simulink model "DC_Model2"  (R2024b)
settings: Solver=VariableStepAuto  StartTime=0.0  StopTime=10  RelTol=1e-6
model workspace (MAT data in the model file):
  B = 0.1
  J = 0.01
  Ke = 0.01
  Kt = 0.01
  L = 0.5
  Req = 1
  Vbat = 24
settings Model: Creator=khalid  LastModifiedBy=khalidwaleed

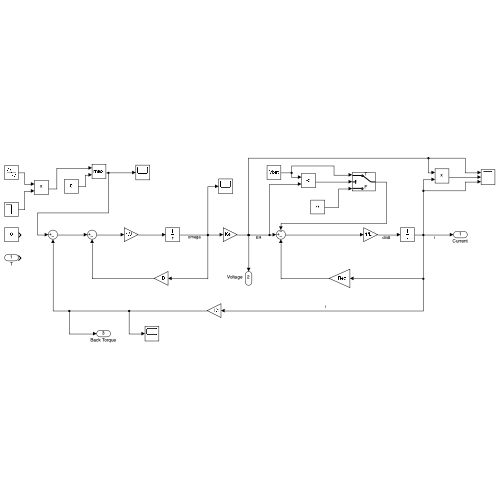
[thumbnail: Simulink's stored preview of the top-level diagram]
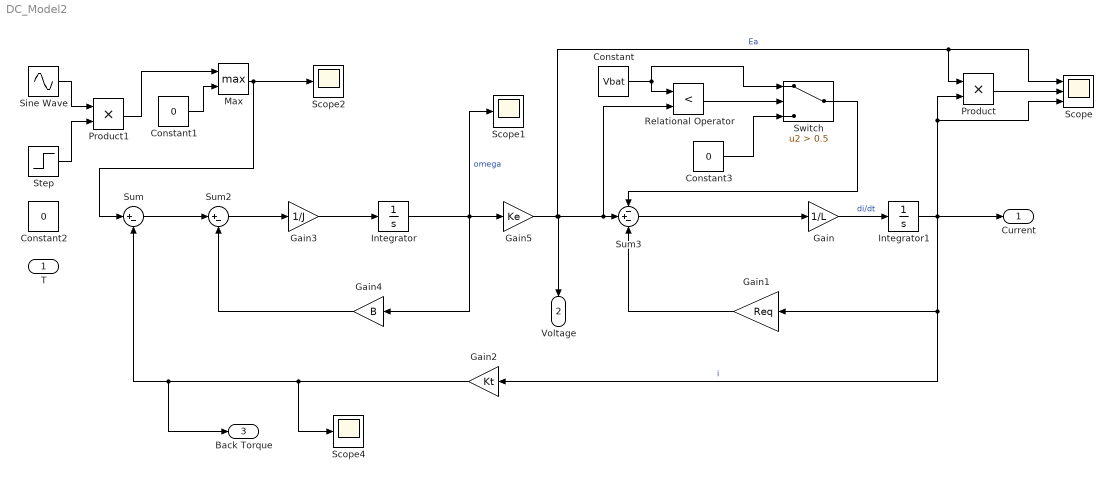
== system DC_Model2 ==
  T : Inport
  Constant : Constant  Value=Vbat
  Constant1 : Constant  Value=0
  Constant2 : Constant  Value=0
  Constant3 : Constant  Value=0
  Gain : Gain  Gain=1/L
  Gain1 : Gain  Gain=Req
  Gain2 : Gain  Gain=Kt
  Gain3 : Gain  Gain=1/J
  Gain4 : Gain  Gain=B
  Gain5 : Gain  Gain=Ke
  Integrator : Integrator
  Integrator1 : Integrator
  Max : MinMax  Function=max  Inputs=2
  Product : Product
  Product1 : Product
  Relational Operator : RelationalOperator  Operator=<  OutDataTypeStr=boolean  RndMeth=Simplest  InputSameDT=off
  Scope : Scope  NumInputPorts=3
  Scope1 : Scope
  Scope2 : Scope
  Scope4 : Scope
  Sine Wave : Sin  Amplitude=1e3  Frequency=20  SampleTime=0
  Step : Step  Time=5  Before=1  After=0  SampleTime=0
  Sum : Sum  Inputs=|+-
  Sum2 : Sum  Inputs=|+-
  Sum3 : Sum  Inputs=-+-
  Switch : Switch  Criteria=u2 > Threshold  Threshold=0.5  SaturateOnIntegerOverflow=off  InputSameDT=off
  Current : Outport
  Voltage : Outport  Port=2
  Back Torque : Outport  Port=3
  wires:
  Gain4/1 -> Sum2/2
  Gain3/1 -> Integrator/1
  Integrator/1 -> Gain5/1, Gain4/1, Scope1/1  "omega"
  Gain2/1 -> Scope4/1, Back Torque/1, Sum/2
  Integrator1/1 -> Gain1/1, Gain2/1, Product/2, Scope/3, Current/1  "i"
  Sum/1 -> Sum2/1
  Gain5/1 -> Relational Operator/2, Sum3/2, Voltage/1, Product/1, Scope/1  "Ea"
  Gain/1 -> Integrator1/1  "di/dt"
  Sum2/1 -> Gain3/1
  Product/1 -> Scope/2
  Sine Wave/1 -> Product1/1
  Step/1 -> Product1/2
  Constant1/1 -> Max/2
  Product1/1 -> Max/1
  Max/1 -> Sum/1, Scope2/1
  Gain1/1 -> Sum3/3
  Sum3/1 -> Gain/1
  Constant/1 -> Switch/1, Relational Operator/1
  Constant3/1 -> Switch/3
  Switch/1 -> Sum3/1
  Relational Operator/1 -> Switch/2
